simulink model "ukol_9_model"  (R2016a)
settings: Solver=VariableStepAuto  StartTime=0.0  StopTime=30  MaxStep=1e-3  RelTol=1e-3
undefined symbols (not defined in the file): A, B, C, D, k1, k2, korekcni_zesileni, L
settings Model: Creator=kuhaj  LastModifiedBy=tomas
settings DataIOCC: LimitDataPoints=on
settings DebuggingCC: AllowSymbolicDim=off
settings ModelReferenceCC: PropagateSignalLabelsOutOfModel=off
settings GRTTargetCC: GeneratePreprocessorConditionals=Use local settings

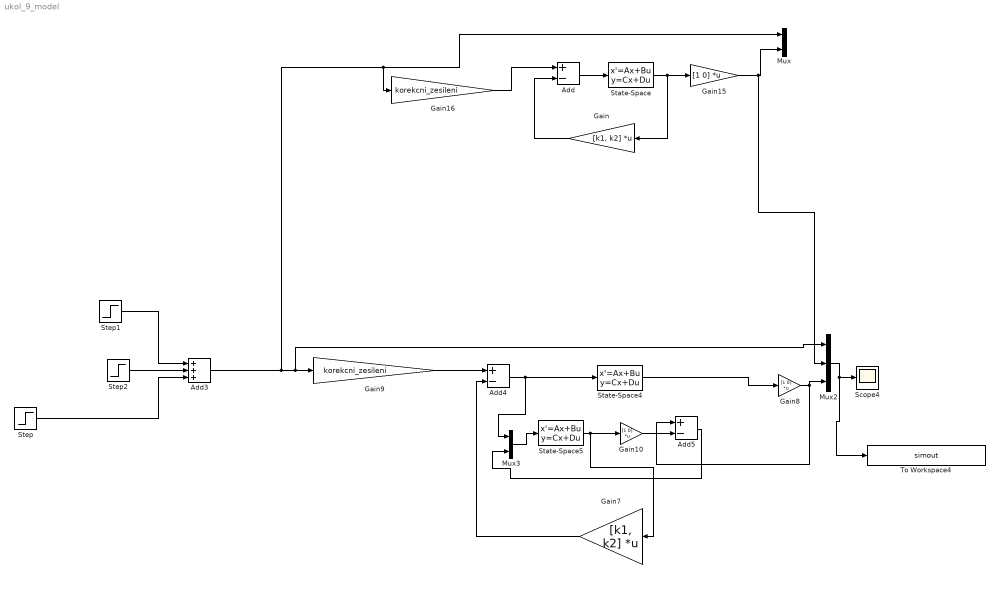
== system ukol_9_model ==
  Add : Sum  Inputs=+-
  Add3 : Sum  Inputs=+++
  Add4 : Sum  Inputs=+-
  Add5 : Sum  Inputs=+-
  Gain : Gain  Gain=[k1, k2]  Multiplication=Matrix(K*u)
  Gain10 : Gain  Gain=[1 0]  Multiplication=Matrix(K*u)
  Gain15 : Gain  Gain=[1 0]  Multiplication=Matrix(K*u)
  Gain16 : Gain  Gain=korekcni_zesileni
  Gain7 : Gain  Gain=[k1, k2]  Multiplication=Matrix(K*u)
  Gain8 : Gain  Gain=[1 0]  Multiplication=Matrix(K*u)
  Gain9 : Gain  Gain=korekcni_zesileni
  Mux : Mux  Inputs=2
  Mux2 : Mux  Inputs=3
  Mux3 : Mux  Inputs=2
  Scope4 : Scope
  State-Space : StateSpace  A=A  B=B  C=C  D=D  X0=0
  State-Space4 : StateSpace  A=A  B=B  C=C  D=D  X0=0
  State-Space5 : StateSpace  A=A  B=[B L]  C=C  D=[0 0; 0 0]  X0=[0.3;-0.2]
  Step : Step  SampleTime=0
  Step1 : Step  Time=10  After=-4  SampleTime=0
  Step2 : Step  Time=20  After=8  SampleTime=0
  To Workspace4 : ToWorkspace  VariableName=simout  SaveFormat=Timeseries  SampleTime=-1
  wires:
  Gain7/1 -> Add4/2
  Add4/1 -> State-Space4/1, Mux3/1
  Gain9/1 -> Add4/1
  Mux2/1 -> Scope4/1, To Workspace4/1
  Gain8/1 -> Mux2/3, Add5/1
  State-Space4/1 -> Gain8/1
  Mux3/1 -> State-Space5/1
  State-Space5/1 -> Gain10/1, Gain7/1
  Gain10/1 -> Add5/2
  Add5/1 -> Mux3/2
  Gain15/1 -> Mux2/2, Mux/2
  Add3/1 -> Gain16/1, Mux/1, Mux2/1, Gain9/1
  Gain16/1 -> Add/1
  Gain/1 -> Add/2
  State-Space/1 -> Gain/1, Gain15/1
  Add/1 -> State-Space/1
  Step2/1 -> Add3/2
  Step1/1 -> Add3/1
  Step/1 -> Add3/3
